simulink model "ex7_model"  (R2021b)
settings: Solver=VariableStepAuto  StartTime=0.0  StopTime=10.0  RelTol=1e-3
values from neighbouring files (symbols this model uses):
  delta_u = 0    [ex2.m]    (also in ex3.m; ex7.m = 1)
  pkp_0 = 89.25    [param.m]
settings Model: Creator=tular  LastModifiedBy=tular

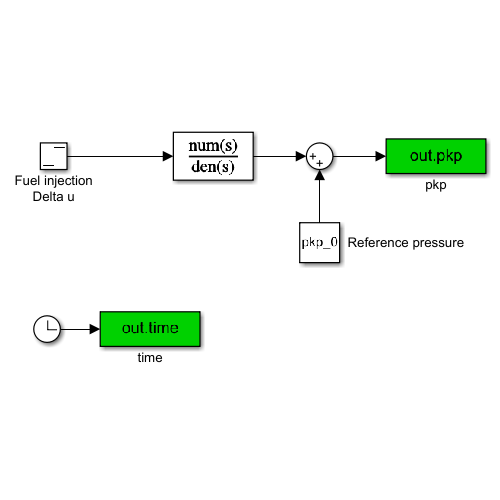
[thumbnail: Simulink's stored preview of the top-level diagram]
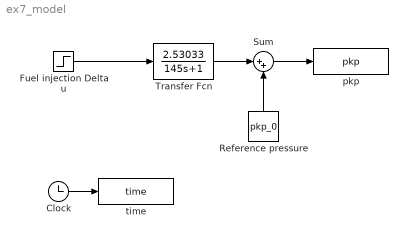
== system ex7_model ==
  Clock : Clock
  Fuel injection Delta u : Step  Time=200  After=delta_u  SampleTime=0
  Reference pressure : Constant  Value=pkp_0
  Sum : Sum  Inputs=|++
  Transfer Fcn : TransferFcn  Numerator=2.53033  Denominator=[145 1]
  pkp : ToWorkspace  VariableName=pkp
      settings: MaxDataPoints=2000
  time : ToWorkspace  VariableName=time
      settings: MaxDataPoints=2000
  wires:
  Fuel injection Delta u/1 -> Transfer Fcn/1
  Transfer Fcn/1 -> Sum/1
  Reference pressure/1 -> Sum/2
  Sum/1 -> pkp/1
  Clock/1 -> time/1
